simulink model "TRUAV_Dynamics_from_GTRS_trim"  (R2022b)
settings: Solver=ode4  StartTime=0.0  StopTime=3  FixedStep=0.004  RelTol=1e-3
values from neighbouring files (symbols this model uses):
  a_sound = 1116.45    [init_0_GTRS_data_Run_this_file.m]
  alpha_F_rad = alpha_F_deg * (pi/180)    [init_Vetical_2_Table.m]
  alpha_F_rad_table = alpha_F_table * (pi/180)    [init_Fuselage_Aero_Table.m]
  alpha_H_rad = alpha_H_deg * (pi/180)    [init_Horizontal_Table.m]
  alpha_HD_rad = alpha_HD_deg * (pi/180)    [init_Horizontal_C_D_Table.m]
  alpha_r0 = 0    [init_0_GTRS_data_Run_this_file.m]
  alpha_WF_epsilon_M_rad = alpha_WF_deg * pi/180    [init_WingWake_Deflection_Table.m]
  alpha_WS_CL_rad = alpha_WS_CL_deg * (pi/180)    [init_Wing_Slide_Table.m]
  b_w = 32.17    [init_0_GTRS_data_Run_this_file.m]
  beta_F_rad = beta_F_deg * (pi/180)    [init_Vetical_2_Table.m]
  beta_LD_rad_table = beta_LD_table * (pi/180)    [init_Fuselage_Aero_Table.m]
  beta_m_epsilon_M_rad = beta_m_deg * pi/180    [init_WingWake_Deflection_Table.m]
  beta_m_rad_cn = beta_m_deg_cn * pi/180    [init_Wing_Free_Table.m]
  beta_M_rad_table = beta_M_table  * (pi/180)    [init_Fuselage_Aero_Table.m]
  beta_m_S_rad = beta_m_S_deg * (pi/180)    [init_Vetical_2_Table.m]
  beta_m_WS_CL_rad = beta_m_WS_CL_deg * (pi/180)    [init_Wing_Slide_Table.m]
  beta_rad_brk = beta_KBR_rad    [init_Vetical_2_Table.m]
  beta_v_rad = beta_v_deg * (pi/180)    [init_Vetical_1_Table.m]
  beta_vD_rad = beta_vD_deg * (pi/180)    [init_Vetical_1_Table.m]
  beta_WF_Cl_rad = beta_W_deg * (pi/180)    [init_Wing_Free_Table.m]
  beta_WF_CL_rad = beta_CL_deg * (pi/180)    [init_Wing_Free_Table.m]
  beta_YlN_rad_table = beta_YlN_table * (pi/180)    [init_Fuselage_Aero_Table.m]
  c_HW = 3.92    [init_0_GTRS_data_Run_this_file.m]
  C_l_beta_CLwp_table = [ ... (first row only)    [init_Wing_Free_Table.m]
  C_l_beta_pro_CLwp_table = [ ... (first row only)    [init_Wing_Free_Table.m]
  C_L_delta_a_table = [0.00316, 0.00396, 0.00476, 0]    [init_Wing_Free_Table.m]
  C_LHB = -0.00422    [init_0_GTRS_data_Run_this_file.m]
  C_lp_C_LWP = -0.774    [init_0_GTRS_data_Run_this_file.m]
  C_m_wp_table = [ ... (first row only)    [init_Wing_Free_Table.m]
  C_MHA = 0    [init_0_GTRS_data_Run_this_file.m]
  C_MHO = 0    [init_0_GTRS_data_Run_this_file.m]
  c_R = 14/12    (= 1.16666666667)    [init_0_GTRS_data_Run_this_file.m]
  c_w = 5.225    [init_0_GTRS_data_Run_this_file.m]
  C_Y_beta = 0    [init_0_GTRS_data_Run_this_file.m]
  CD0_high_Mach_data = [0.0177, 0.0178, 0.0179, 0.0405]    [init_Wing_Free_Table.m]
  CD_4D_table = zeros(49, 4, 2, 4)    [init_Wing_Slide_Table.m]
  CDH_2D_table = zeros(length(alpha_HD_deg), length(mach_vec))    [init_Horizontal_C_D_Table.m]
  CDV_2D_table = zeros(length(beta_vD_deg), length(mach_vec))    [init_Vetical_1_Table.m]
  CL_4D_table = zeros(49, 4, 2, 4)    [init_Wing_Slide_Table.m]
  CLH_3D_table = zeros(length(alpha_H_deg), length(delta_e_deg), length(mach_vec))    [init_Horizontal_Table.m]
  CYV_3D_table = zeros(length(beta_v_deg), length(delta_r_deg), length(mach_vec))    [init_Vetical_1_Table.m]
  D_alpha_table = [D_part1, D_part2, D_part3, D_part4]    [init_Fuselage_Aero_Table.m]
  D_beta_table = [ fliplr(D_beta_half(2:end)),  D_beta_half]    [init_Fuselage_Aero_Table.m]
  D_ke = 0.24    [init_0_GTRS_data_Run_this_file.m]
  D_Kr = 0.24    [init_0_GTRS_data_Run_this_file.m]    (also in init_Vetical_1_Table.m)
  DBFO = -1.56    [init_0_GTRS_data_Run_this_file.m]
  delta_e_rad = delta_e_deg * (pi/180)    [init_Horizontal_Table.m]
  delta_r_deg = [-20, -15, 0, 15, 20]    [init_Vetical_1_Table.m]
  DLANG = -0.5    [init_0_GTRS_data_Run_this_file.m]
  epsilon_W_table = permute(epsilon_W_3D, [3, 1, 2])    [init_WingWake_Deflection_Table.m]
  flap_rad = flap_deg * (pi/180)    [init_Wing_Free_Table.m]    (also in init_Wing_Slide_Table.m)
  ft2m = 0.3048    [init_0_GTRS_data_Run_this_file.m]
  h_HW = [-0.5838, 0.01158, 0.5967, 0.002547,-2.2519]    [init_0_GTRS_data_Run_this_file.m]
  I_b = 102.5    [init_0_GTRS_data_Run_this_file.m]
  i_H = 0    [init_0_GTRS_data_Run_this_file.m]
  i_v = 0    [init_0_GTRS_data_Run_this_file.m]
  i_w = 0    [init_0_GTRS_data_Run_this_file.m]
  in2ft = 1/12    (= 0.0833333333333)    [init_0_GTRS_data_Run_this_file.m]
  Ixx = 52795    [init_0_GTRS_data_Run_this_file.m]
  Ixz = 1234    [init_0_GTRS_data_Run_this_file.m]
  Iyy = 21360    [init_0_GTRS_data_Run_this_file.m]
  Izz = 66335    [init_0_GTRS_data_Run_this_file.m]
  K1delta_data = [ ... (first row only)    [init_Wing_Free_Table.m]
  K_coeffs = [1.6 0]    [init_0_GTRS_data_Run_this_file.m]
  K_FWDF = -0.0035    [init_0_GTRS_data_Run_this_file.m]
  K_FWO = 1.4    [init_0_GTRS_data_Run_this_file.m]
  K_HNU = 0.8    [init_0_GTRS_data_Run_this_file.m]
  K_vNU = 1    [init_Vetical_1_Table.m]
  KBR_table = KBR_table_full    [init_Vetical_2_Table.m]
  Kn_delta_data = [ ... (first row only)    [init_Wing_Free_Table.m]
  Kno_delta_data = [ ... (first row only)    [init_Wing_Free_Table.m]
  L_alpha_table = [L_part1, L_part2, L_part3, L_part4]    [init_Fuselage_Aero_Table.m]
  L_beta_table = [ fliplr(L_beta_half(2:end)),  L_beta_half]    [init_Fuselage_Aero_Table.m]
  l_beta_table = [l_beta_neg, l_beta_pos]    [init_Fuselage_Aero_Table.m]
  L_n = 4.667    [init_0_GTRS_data_Run_this_file.m]
  lambda_w = -6.5*deg2rad    (= -0.11344640138)    [init_0_GTRS_data_Run_this_file.m]
  LBFO = -7.23    [init_0_GTRS_data_Run_this_file.m]
  LLANG = 0    [init_0_GTRS_data_Run_this_file.m]
  m2ft = 1/ft2m    (= 3.28083989501)    [init_0_GTRS_data_Run_this_file.m]
  M_alpha_table = [M_part1, M_part2, M_part3, M_part4]    [init_Fuselage_Aero_Table.m]
  M_beta_table = [ fliplr(M_beta_half(2:end)), M_beta_half]    [init_Fuselage_Aero_Table.m]
  Mach_brk = [0.2, 0.4, 0.5, 0.6]    [init_Wing_Free_Table.m]
  mach_vec = [0.2, 0.4, 0.5, 0.6]    [init_Horizontal_C_D_Table.m]    (also in init_Horizontal_Table.m; init_Vetical_1_Table.m)
  mass = 403.7    [init_0_GTRS_data_Run_this_file.m]
  mast_rad = mast_deg * pi/180    [init_Wing_Free_Table.m]
  MBFO = 66.5    [init_0_GTRS_data_Run_this_file.m]
  Mn_X_ke = [0 0.2 0.4 0.5 0.6 0.7]    [init_Horizontal_Table.m]
  N_beta_table = [N_beta_neg, N_beta_pos]    [init_Fuselage_Aero_Table.m]
  pos_x_CG = 300    [init_0_GTRS_data_Run_this_file.m]
  pos_x_H = 300    [init_0_GTRS_data_Run_this_file.m]
  pos_x_HW = 560    [init_0_GTRS_data_Run_this_file.m]
  pos_x_Nac = 291.7    [init_0_GTRS_data_Run_this_file.m]
  pos_x_V = 570    [init_0_GTRS_data_Run_this_file.m]
  pos_x_W = 291.7    [init_0_GTRS_data_Run_this_file.m]
  pos_y_CG = 0    [init_0_GTRS_data_Run_this_file.m]
  pos_y_H = 193    [init_0_GTRS_data_Run_this_file.m]
  pos_y_HW = 0    [init_0_GTRS_data_Run_this_file.m]
  pos_y_Nac = 193    [init_0_GTRS_data_Run_this_file.m]
  pos_y_V = 115.69    [init_0_GTRS_data_Run_this_file.m]
  pos_y_W = 96.6    [init_0_GTRS_data_Run_this_file.m]
  pos_z_CG = 81.65    [init_0_GTRS_data_Run_this_file.m]
  pos_z_H = 100    [init_0_GTRS_data_Run_this_file.m]
  pos_z_HW = 103    [init_0_GTRS_data_Run_this_file.m]
  pos_z_Nac = 118    [init_0_GTRS_data_Run_this_file.m]
  pos_z_V = 77    [init_0_GTRS_data_Run_this_file.m]
  pos_z_W = 96    [init_0_GTRS_data_Run_this_file.m]
  R = 12.5    [init_0_GTRS_data_Run_this_file.m]
  rho = 0.002376    [init_0_GTRS_data_Run_this_file.m]
  s_HW = 50.25    [init_0_GTRS_data_Run_this_file.m]
  S_max = 56    [init_0_GTRS_data_Run_this_file.m]
  S_v = 20.25    [init_0_GTRS_data_Run_this_file.m]
  S_w = 181    [init_0_GTRS_data_Run_this_file.m]
  Sidewash_4D = zeros(length(alpha_F_deg), length(beta_F_deg), length(beta_m_S_deg), length(delta_F_S_deg))    [init_Vetical_2_Table.m]
  slugft2kgm = 1.35582    [init_0_GTRS_data_Run_this_file.m]
  tau_e = 0.518    [init_0_GTRS_data_Run_this_file.m]
  tau_r = 0.27    [init_0_GTRS_data_Run_this_file.m]    (also in init_Vetical_1_Table.m)
  theta_0_R = 0.750    (= 0.75)    [init_0_GTRS_data_Run_this_file.m]
  theta_0_W = 1.187    [init_0_GTRS_data_Run_this_file.m]
  theta_twist = -41*deg2rad    (= -0.715584993318)    [init_0_GTRS_data_Run_this_file.m]
  u_max = 1181/12    (= 98.4166666667)    [init_0_GTRS_data_Run_this_file.m]
  ... (+3 more)
undefined symbols (not defined in the file or in its folder): beta_m_rad, F, Light, MIL, sigbuilder_block, tilt_cmd
libraries: simulink x2, sharedtransform x2, aerolibasang x2, aerolibwind2 x1
(part 1 of 4)
settings Model: PacingRate=10  Creator=57178  LastModifiedBy=57178

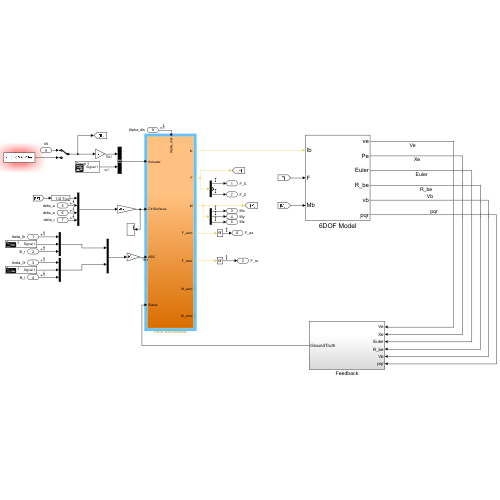
[thumbnail: Simulink's stored preview of the top-level diagram]
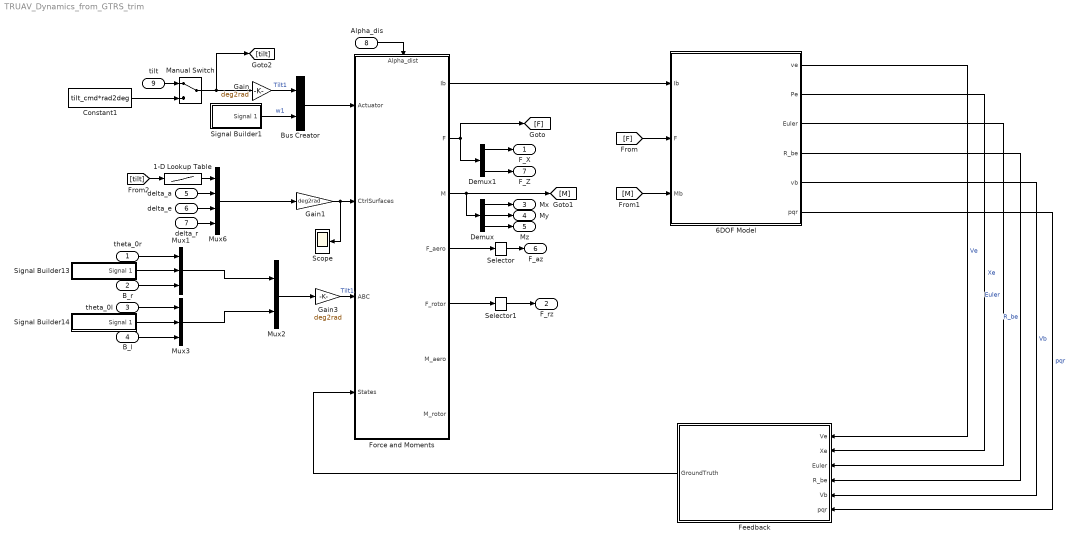
== system TRUAV_Dynamics_from_GTRS_trim ==
  theta_0r : Inport
  B_r : Inport  Port=2
  theta_0l : Inport  Port=3
  B_l : Inport  Port=4
  delta_a : Inport  Port=5
  delta_e : Inport  Port=6
  delta_r : Inport  Port=7
  Alpha_dis : Inport  Port=8
  tilt : Inport  Port=9
  1-D Lookup Table : Lookup_n-D  NumberOfTableDimensions=1  BreakpointsForDimension1=[0, 15, 30, 60, 90]  Table=[75, 75, 50, 10, 0]  InternalRulePriority=Speed  RndMeth=Simplest
  6DOF Model : Subsystem
  Bus Creator : BusCreator  Inputs=2
  Constant1 : Constant  Value=tilt_cmd*rad2deg
  Demux : Demux  Outputs=3
  Demux1 : Demux  Outputs=3
  Feedback : Subsystem
  Force and Moments : Subsystem
      settings: PortSchema="{\"entries\":[{\"content\":{\"sides\":[{\"content\":{\"connectorIds\":[\"In1\",\"In2\",\"In3\",\"In4\"]},\"type\":\"ConnectorPlacement.EquallySpacedRectSide\",\"uuid\":\"14175658-dd1e-49e4-b43b-ea4e1e064656\"},{\"content\":{\"connectorIds\":[\"Out1\",\"Out2\",\"Out3\",\"Out4\",\"Out5\",\"Out6\",\"Out7\"],\"side\":\"RIGHT\"},\"type\":\"ConnectorPlacement.EquallySpacedRectSide\",\"uuid\":\"2cac6120-f4ef-4ea4-82cf-37ab6ff67795\"},{\"content\":{\"connectorIds\":[\"In5\"],\"side\":\"TOP\"},\"type\":\"ConnectorPlacement.EquallySpacedRectSide\",\"uuid\":\"384cf1cc-0caa-4cb0-88f0-d3cb4556450a\"}]},\"type\":\"ConnectorPlacement.EquallySpacedConnector\",\"uuid\":\"6851ebde-8421-46a5-9721-7873d89ee264\"}],\"packageUris\":[\"http://schema.mathworks.com/mf0/Connector/R2020b\"],\"version\":\"1.0\"}"
  Gain : Gain  Gain=deg2rad
  Gain1 : Gain  Gain=deg2rad
  Gain3 : Gain  Gain=deg2rad
  Manual Switch : ManualSwitch
  Mux1 : Mux  Inputs=3
  Mux2 : Mux  Inputs=2
  Mux3 : Mux  Inputs=3
  Mux6 : Mux
  Scope : Scope
  Selector : Selector  InputPortWidth=3  IndexOptions=Index vector (dialog)  Indices=[3]  OutputSizes=1
  Selector1 : Selector  InputPortWidth=3  IndexOptions=Index vector (dialog)  Indices=[3]  OutputSizes=1
  Signal Builder1 : Subsystem  Tag=STV Subsys  LoadFcn=sigbuilder_block('load');  StartFcn=sigbuilder_block('start');  StopFcn=sigbuilder_block('stop');  ClipboardFcn=sigbuilder_block('clipboard');  mask(Sigbuilder block){tuvar=[0:10]}
      mask help: Simulink:masks:SigbuilderBlock_MD
      mask init:
      | if ~strcmp(get_param(bdroot(gcbh),'SimulationStatus'),'stopped') tuvar = sigbuilder_block('maskInit'); end
      settings: CopyFcn=sigbuilder_block('copy');  DeleteFcn=sigbuilder_block('delete');  ModelCloseFcn=sigbuilder_block('modelClose');  PreSaveFcn=sigbuilder_block('preSave');  PauseFcn=sigbuilder_block('pause');  ContinueFcn=sigbuilder_block('continue');  NameChangeFcn=sigbuilder_block('namechange');  OpenFcn=sigbuilder_block('open',[437.6 199.2 550.4 400 ]);  CloseFcn=sigbuilder_block('close');
      mask Display: plot(0, 0, 100, 100,[2, 2, 32, 32, 2], [68, 8, 8, 68, 68],[32, 2], [38, 38], [32, 19, 2],[53, 60, 44], [32, 17, 17, 2],[16, 16, 31, 31]);txt = getActiveGroup(gcbh);text(2, 100, txt,'verticalAlignment', 'top');
  Signal Builder13 : Subsystem  Tag=STV Subsys  LoadFcn=sigbuilder_block('load');  StartFcn=sigbuilder_block('start');  StopFcn=sigbuilder_block('stop');  ClipboardFcn=sigbuilder_block('clipboard');  mask(Sigbuilder block){tuvar=[0:10]}
      mask help: Simulink:masks:SigbuilderBlock_MD
      mask init:
      | if ~strcmp(get_param(bdroot(gcbh),'SimulationStatus'),'stopped') tuvar = sigbuilder_block('maskInit'); end
      settings: CopyFcn=sigbuilder_block('copy');  DeleteFcn=sigbuilder_block('delete');  ModelCloseFcn=sigbuilder_block('modelClose');  PreSaveFcn=sigbuilder_block('preSave');  PauseFcn=sigbuilder_block('pause');  ContinueFcn=sigbuilder_block('continue');  NameChangeFcn=sigbuilder_block('namechange');  OpenFcn=sigbuilder_block('open',[-1344 -173.143 550.286 399.857 ]);  CloseFcn=sigbuilder_block('close');
      mask Display: plot(0, 0, 100, 100,[2, 2, 32, 32, 2], [68, 8, 8, 68, 68],[32, 2], [38, 38], [32, 19, 2],[53, 60, 44], [32, 17, 17, 2],[16, 16, 31, 31]);txt = getActiveGroup(gcbh);text(2, 100, txt,'verticalAlignment', 'top');
  Signal Builder14 : Subsystem  Tag=STV Subsys  LoadFcn=sigbuilder_block('load');  StartFcn=sigbuilder_block('start');  StopFcn=sigbuilder_block('stop');  ClipboardFcn=sigbuilder_block('clipboard');  mask(Sigbuilder block){tuvar=[0:10]}
      mask help: Simulink:masks:SigbuilderBlock_MD
      mask init:
      | if ~strcmp(get_param(bdroot(gcbh),'SimulationStatus'),'stopped') tuvar = sigbuilder_block('maskInit'); end
      settings: CopyFcn=sigbuilder_block('copy');  DeleteFcn=sigbuilder_block('delete');  ModelCloseFcn=sigbuilder_block('modelClose');  PreSaveFcn=sigbuilder_block('preSave');  PauseFcn=sigbuilder_block('pause');  ContinueFcn=sigbuilder_block('continue');  NameChangeFcn=sigbuilder_block('namechange');  OpenFcn=sigbuilder_block('open',[-1344 -173.143 550.286 399.857 ]);  CloseFcn=sigbuilder_block('close');
      mask Display: plot(0, 0, 100, 100,[2, 2, 32, 32, 2], [68, 8, 8, 68, 68],[32, 2], [38, 38], [32, 19, 2],[53, 60, 44], [32, 17, 17, 2],[16, 16, 31, 31]);txt = getActiveGroup(gcbh);text(2, 100, txt,'verticalAlignment', 'top');
  F_X : Outport
  F_rz : Outport  Port=2
  Mx : Outport  Port=3
  My : Outport  Port=4
  Mz : Outport  Port=5
  F_az : Outport  Port=6
  F_Z : Outport  Port=7
  wires:
  6DOF Model/5(vb) -> Feedback/5(Vb)  "Vb"
  6DOF Model/4(R_be) -> Feedback/4(R_be)  "R_be"
  6DOF Model/2(Pe) -> Feedback/2(Xe)  "Xe"
  [M] -> 6DOF Model/3(Mb)
  [F] -> 6DOF Model/2(F)
  6DOF Model/3(Euler) -> Feedback/3(Euler)  "Euler"
  6DOF Model/6(pqr) -> Feedback/6(pqr)  "pqr"
  Feedback/1(GroundTruth) -> Force and Moments/4(States)
  6DOF Model/1(ve) -> Feedback/1(Ve)  "Ve"
  Force and Moments/2(F) -> Demux1/1, [F]
  Force and Moments/3(M) -> Demux/1, [M]
  Gain/1 -> Bus Creator/1  "Tilt1"
  Signal Builder1/1(Signal 1) -> Bus Creator/2  "w1"
  Bus Creator/1 -> Force and Moments/1(Actuator)
  Mux6/1 -> Gain1/1
  Mux2/1 -> Gain3/1
  Manual Switch/1 -> [tilt], Gain/1
  Gain3/1 -> Force and Moments/3(ABC)  "Tilt1"
  Gain1/1 -> Scope/1, Force and Moments/2(CtrlSurfaces)
  Force and Moments/1(Ib) -> 6DOF Model/1(Ib)
  theta_0r/1 -> Mux1/1
  Signal Builder13/1(Signal 1) -> Mux1/2
  B_r/1 -> Mux1/3
  theta_0l/1 -> Mux3/1
  Signal Builder14/1(Signal 1) -> Mux3/2
  B_l/1 -> Mux3/3
  Mux1/1 -> Mux2/1
  Mux3/1 -> Mux2/2
  1-D Lookup Table/1 -> Mux6/1
  delta_r/1 -> Mux6/4
  delta_e/1 -> Mux6/3
  delta_a/1 -> Mux6/2
  Demux/1 -> Mx/1
  Demux/3 -> Mz/1
  Demux/2 -> My/1
  Demux1/1 -> F_X/1
  Demux1/3 -> F_Z/1
  Alpha_dis/1 -> Force and Moments/5(Alpha_dist)
  Force and Moments/4(F_aero) -> Selector/1
  Selector/1 -> F_az/1
  Selector1/1 -> F_rz/1
  [tilt] -> 1-D Lookup Table/1
  Force and Moments/5(F_rotor) -> Selector1/1
  Constant1/1 -> Manual Switch/2
  tilt/1 -> Manual Switch/1

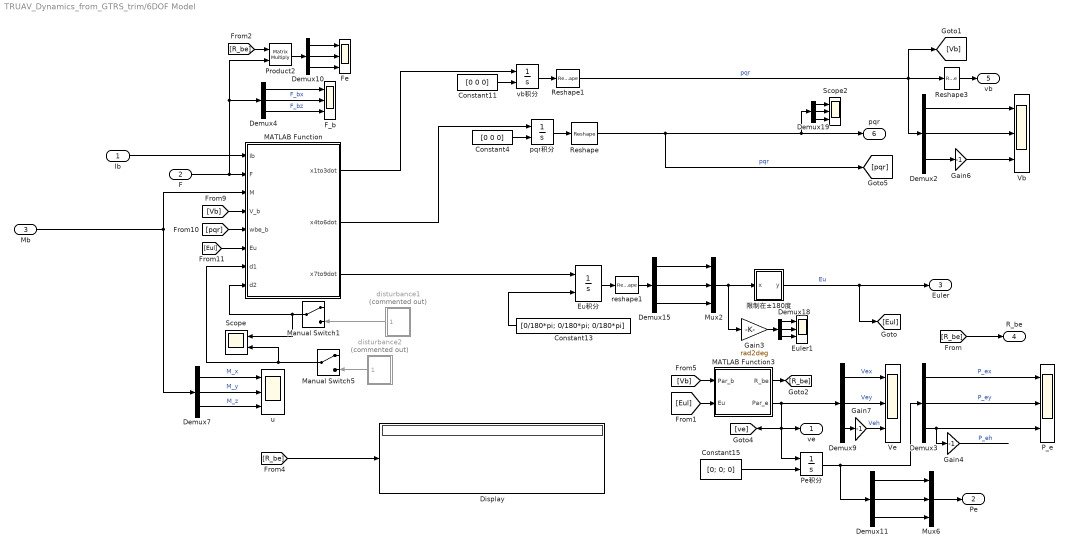
== system TRUAV_Dynamics_from_GTRS_trim/6DOF Model ==
  Ib : Inport
  F : Inport  Port=2
  Mb : Inport  Port=3
  Constant11 : Constant  Value=[0 0 0]
  Constant13 : Constant  Value=[0/180*pi; 0/180*pi; 0/180*pi]
  Constant15 : Constant  Value=[0; 0; 0]
  Constant4 : Constant  Value=[0 0 0]
  Demux{2..4,7,9..11,15,18..19} (10 alike) : Demux  Outputs=3
  Display : Display
  Euler1 : Scope  NumInputPorts=3
  Eu积分 : Integrator  InitialConditionSource=external
  F_b : Scope  NumInputPorts=3
  Fe : Scope  NumInputPorts=3
  Gain3 : Gain  Gain=rad2deg
  Gain4 : Gain  Gain=-1
  Gain6 : Gain  Gain=-1
  Gain7 : Gain  Gain=-1
  MATLAB Function : MATLAB Function  TreatAsAtomicUnit=on
  MATLAB Function3 : MATLAB Function  TreatAsAtomicUnit=on
  Manual Switch1 : ManualSwitch
  Manual Switch5 : ManualSwitch
  Mux2 : Mux  Inputs=3
  Mux6 : Mux  Inputs=3
  P_e : Scope  NumInputPorts=3
  Pe积分 : Integrator  InitialConditionSource=external
  Product2 : Product  Multiplication=Matrix(*)
  Reshape : Reshape  OutputDimensionality=Customize  OutputDimensions=[3,1]
  Reshape1 : Reshape  OutputDimensionality=Customize  OutputDimensions=[3,1]
  Reshape3 : Reshape  OutputDimensionality=Column vector (2-D)
  Scope : Scope  NumInputPorts=2
  Scope2 : Scope  NumInputPorts=3
  Vb : Scope  NumInputPorts=3
  Ve : Scope  NumInputPorts=3
  disturbance1 : Subsystem  Commented=on
  disturbance2 : Subsystem  Commented=on
  pqr积分 : Integrator  InitialConditionSource=external
  reshape1 : Reshape  OutputDimensionality=Customize  OutputDimensions=[3,1]
  u : Scope  NumInputPorts=3
  vb积分 : Integrator  InitialConditionSource=external
  限制在±180度 : MATLAB Function  TreatAsAtomicUnit=on
  ve : Outport
  Pe : Outport  Port=2
  Euler : Outport  Port=3  VectorParamsAs1DForOutWhenUnconnected=off
  R_be : Outport  Port=4  VectorParamsAs1DForOutWhenUnconnected=off
  vb : Outport  Port=5  VectorParamsAs1DForOutWhenUnconnected=off
  pqr : Outport  Port=6  VectorParamsAs1DForOutWhenUnconnected=off
  wires:
  Demux3/3 -> P_e/3, Gain4/1
  Demux3/1 -> P_e/1  "P_ex"
  [Eul] -> MATLAB Function3/2(Eu)
  MATLAB Function3/2(Par_e) -> Pe积分/1, [ve], ve/1, Demux9/1
  Demux9/3 -> Gain7/1
  Demux9/1 -> Ve/1  "Vex"
  Demux9/2 -> Ve/2  "Vey"
  Mb/1 -> MATLAB Function/3(M), Demux7/1
  Demux7/3 -> u/3  "M_z"
  Demux7/1 -> u/1  "M_x"
  Demux7/2 -> u/2  "M_y"
  限制在±180度/1(y) -> [Eul], Euler/1  "Eu"
  Manual Switch1/1 -> MATLAB Function/8(d2), Scope/1
  Demux4/1 -> F_b/1  "F_bx"
  Demux4/2 -> F_b/2
  Demux4/3 -> F_b/3  "F_bz"
  Demux2/3 -> Gain6/1
  Demux2/2 -> Vb/2
  Demux2/1 -> Vb/1
  Demux15/3 -> Mux2/3
  Demux15/1 -> Mux2/1
  Mux2/1 -> Gain3/1, 限制在±180度/1(x)
  pqr积分/1 -> Reshape/1
  MATLAB Function/1(x1to3dot) -> vb积分/1
  reshape1/1 -> Demux15/1
  Eu积分/1 -> reshape1/1
  MATLAB Function/3(x7to9dot) -> Eu积分/1
  Constant4/1 -> pqr积分/2
  Constant11/1 -> vb积分/2
  vb积分/1 -> Reshape1/1
  disturbance1/1(Out1) -> Manual Switch1/2
  Demux18/2 -> Euler1/2
  Demux18/3 -> Euler1/3
  Demux18/1 -> Euler1/1
  Gain3/1 -> Demux18/1
  Demux19/3 -> Scope2/3
  Demux19/1 -> Scope2/1
  Demux19/2 -> Scope2/2
  Constant15/1 -> Pe积分/2
  MATLAB Function3/1(R_be) -> [R_be]
  [R_be] -> R_be/1
  Demux3/2 -> P_e/2  "P_ey"
  Gain4/1 -> ?  "P_eh"
  [R_be] -> Display/1
  MATLAB Function/2(x4to6dot) -> pqr积分/1
  Constant13/1 -> Eu积分/2
  [Vb] -> MATLAB Function3/1(Par_b)
  Mux6/1 -> Pe/1
  Demux11/2 -> Mux6/2
  Pe积分/1 -> Demux11/1, Demux3/1
  Demux11/3 -> Mux6/3
  Demux11/1 -> Mux6/1
  Demux15/2 -> Mux2/2
  Demux10/3 -> Fe/3
  Product2/1 -> Demux10/1
  Demux10/2 -> Fe/2
  Demux10/1 -> Fe/1
  [R_be] -> Product2/1
  F/1 -> MATLAB Function/2(F), Product2/2, Demux4/1
  [Vb] -> MATLAB Function/4(V_b)
  [pqr] -> MATLAB Function/5(wbe_b)
  [Eul] -> MATLAB Function/6(Eu)
  Manual Switch5/1 -> MATLAB Function/7(d1), Scope/2
  Gain6/1 -> Vb/3
  Gain7/1 -> Ve/3  "Veh"
  Ib/1 -> MATLAB Function/1(Ib)
  disturbance2/1(Out1) -> Manual Switch5/2
  Reshape1/1 -> Demux2/1, Reshape3/1, [Vb]  "pqr"
  Reshape3/1 -> vb/1
  Reshape/1 -> Demux19/1, pqr/1, [pqr]  "pqr"

== system TRUAV_Dynamics_from_GTRS_trim/Feedback ==
  Ve : Inport
  Xe : Inport  Port=2
  Euler : Inport  Port=3
  R_be : Inport  Port=4
  Vb : Inport  Port=5
  pqr : Inport  Port=6
  Direction Cosine Matrix to Quaternions : sharedtransform/Direction Cosine Matrix  to Quaternions  aMode=0  action=None  tolerance=eps(2)
      settings: LibrarySourceBlock=|
      | aerolibtransform2/Direction Cosine Matrix
      | to Quaternions
  MATLAB Function1 : MATLAB Function  TreatAsAtomicUnit=on
  Reshape : Reshape  OutputDimensionality=Column vector (2-D)
  Reshape1 : Reshape  OutputDimensionality=Column vector (2-D)
  Selector : Selector  InputPortWidth=3  IndexOptions=Index vector (dialog)  Indices=[3 2 1]  OutputSizes=1
  Transpose : Math  Operator=transpose
  Bus Element Out : Outport  PortName=GroundTruth  Element=course
  Bus Element Out1 : Outport  PortName=GroundTruth  Element=gndspeed
  Bus Element Out3 : Outport  PortName=GroundTruth  Element=Xe
  Bus Element Out4 : Outport  PortName=GroundTruth  Element=Ve
  Bus Element Out7 : Outport  PortName=GroundTruth  Element=R_be
  Bus Element Out8 : Outport  PortName=GroundTruth  Element=q
  Bus Element Out9 : Outport  PortName=GroundTruth  Element=pqr
  Bus Element Out6 : Outport  PortName=GroundTruth  Element=Vb
  Bus Element Out5 : Outport  PortName=GroundTruth  Element=Euler
  Bus Element Out13 : Outport  PortName=GroundTruth  Element=ypr
  Bus Element Out14 : Outport  PortName=GroundTruth  Element=Ve_ground
  wires:
  Reshape1/1 -> Bus Element Out6/1
  Reshape/1 -> Bus Element Out5/1, Selector/1
  Selector/1 -> Bus Element Out13/1
  pqr/1 -> Bus Element Out9/1
  Direction Cosine Matrix to Quaternions/1 -> Bus Element Out8/1  "q"
  Vb/1 -> Reshape1/1
  Euler/1 -> Reshape/1
  Xe/1 -> Bus Element Out3/1
  MATLAB Function1/2(gndSpeed) -> Bus Element Out1/1  "gndspeed"
  MATLAB Function1/1(course) -> Bus Element Out/1  "course"
  Ve/1 -> MATLAB Function1/1(vxyz), Bus Element Out4/1, Bus Element Out14/1
  R_be/1 -> Transpose/1, Bus Element Out7/1
  Transpose/1 -> Direction Cosine Matrix to Quaternions/1

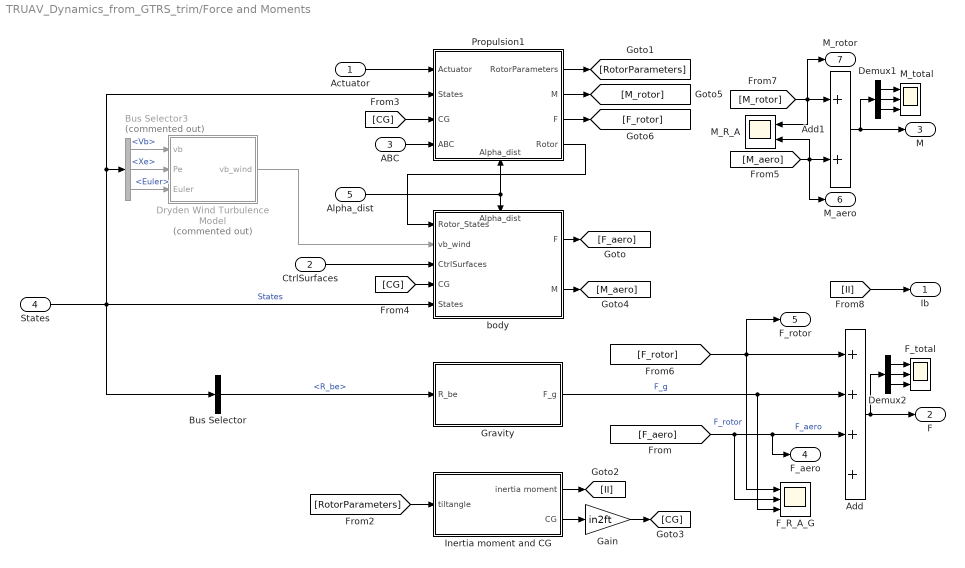
== system TRUAV_Dynamics_from_GTRS_trim/Force and Moments ==
  Actuator : Inport
  CtrlSurfaces : Inport  Port=2
  ABC : Inport  Port=3
  States : Inport  Port=4
  Alpha_dist : Inport  Port=5
  Add : Sum  Inputs=++++
  Add1 : Sum
  Bus Selector : BusSelector  OutputSignals=R_be
  Bus Selector3 : BusSelector  Commented=on  OutputSignals=Vb,Xe,Euler
  Demux1 : Demux  Outputs=3
  Demux2 : Demux  Outputs=3
  "Dryden Wind Turbulence Model " : Subsystem  Commented=on
  F_R_A_G : Scope  NumInputPorts=3
  F_total : Scope  NumInputPorts=3
  Gain : Gain  Gain=in2ft
  Gravity : Subsystem
  Inertia moment and CG : Subsystem
  M_R_A : Scope  NumInputPorts=2
  M_total : Scope  NumInputPorts=3
  Propulsion1 : Subsystem
      settings: PortSchema="{\"entries\":[{\"content\":{\"sides\":[{\"content\":{\"connectorIds\":[\"In1\",\"In2\",\"In3\",\"In4\"]},\"type\":\"ConnectorPlacement.EquallySpacedRectSide\",\"uuid\":\"6f2dbf48-690a-489c-8000-4c6cd685a3c0\"},{\"content\":{\"connectorIds\":[\"Out1\",\"Out2\",\"Out3\",\"Out4\"],\"side\":\"RIGHT\"},\"type\":\"ConnectorPlacement.EquallySpacedRectSide\",\"uuid\":\"c26906ca-dfe8-4bd8-a446-638a7a033ba1\"},{\"content\":{\"connectorIds\":[],\"side\":\"TOP\"},\"type\":\"ConnectorPlacement.EquallySpacedRectSide\",\"uuid\":\"7c8468f6-8fb2-4195-8877-8a49a6dfa1f5\"},{\"content\":{\"connectorIds\":[\"In5\"],\"side\":\"BOTTOM\"},\"type\":\"ConnectorPlacement.EquallySpacedRectSide\",\"uuid\":\"9f190dd0-766f-495f-83f9-cb048c56ad4a\"}]},\"type\":\"ConnectorPlacement.EquallySpacedConnector\",\"uuid\":\"be6e6569-2cab-4e42-86d9-8b4e7133f4ae\"}],\"packageUris\":[\"http://schema.mathworks.com/mf0/Connector/R2020b\"],\"version\":\"1.0\"}"
  body : Subsystem
      settings: PortSchema="{\"entries\":[{\"content\":{\"sides\":[{\"content\":{\"connectorIds\":[\"In1\",\"In2\",\"In3\",\"In4\",\"In5\"]},\"type\":\"ConnectorPlacement.EquallySpacedRectSide\",\"uuid\":\"57bbf977-6343-4159-b754-e5d2e9fd81d9\"},{\"content\":{\"connectorIds\":[\"Out1\",\"Out2\"],\"side\":\"RIGHT\"},\"type\":\"ConnectorPlacement.EquallySpacedRectSide\",\"uuid\":\"304a29c9-3542-4502-b32f-72f6699ccbb9\"},{\"content\":{\"connectorIds\":[\"In6\"],\"side\":\"TOP\"},\"type\":\"ConnectorPlacement.EquallySpacedRectSide\",\"uuid\":\"a47e5583-e12a-44fe-beb4-06c0064b8ef5\"},{\"content\":{\"connectorIds\":[],\"side\":\"BOTTOM\"},\"type\":\"ConnectorPlacement.EquallySpacedRectSide\",\"uuid\":\"46911a4c-96f8-437e-85a1-c5a709ead67b\"}]},\"type\":\"ConnectorPlacement.EquallySpacedConnector\",\"uuid\":\"5ab3fb2f-b501-478f-a319-bc831e44ee3d\"}],\"packageUris\":[\"http://schema.mathworks.com/mf0/Connector/R2020b\"],\"version\":\"1.0\"}"
  Ib : Outport
  F : Outport  Port=2
  M : Outport  Port=3
  F_aero : Outport  Port=4
  F_rotor : Outport  Port=5
  M_aero : Outport  Port=6
  M_rotor : Outport  Port=7
  wires:
  Gravity/1(F_g) -> F_R_A_G/3, Add/2  "F_g"
  States/1 -> Bus Selector/1, body/5(States), Propulsion1/2(States), Bus Selector3/1  "States"
  [F_aero] -> F_R_A_G/2, F_aero/1, Add/3  "F_aero"
  Bus Selector3/2 -> "Dryden Wind Turbulence Model "/2(Pe)  "<Xe>"
  Bus Selector3/3 -> "Dryden Wind Turbulence Model "/3(Euler)  "<Euler>"
  Bus Selector/1 -> Gravity/1(R_be)  "<R_be>"
  [RotorParameters] -> Inertia moment and CG/1(tiltangle)
  Inertia moment and CG/1(inertia moment) -> [II]
  Inertia moment and CG/2(CG) -> Gain/1
  [CG] -> Propulsion1/3(CG)
  Propulsion1/1(RotorParameters) -> [RotorParameters]
  Actuator/1 -> Propulsion1/1(Actuator)
  [CG] -> body/4(CG)
  Gain/1 -> [CG]
  CtrlSurfaces/1 -> body/3(CtrlSurfaces)
  Propulsion1/4(Rotor) -> body/1(Rotor_States)
  body/1(F) -> [F_aero]
  body/2(M) -> [M_aero]
  Propulsion1/2(M) -> [M_rotor]
  Propulsion1/3(F) -> [F_rotor]
  [F_rotor] -> Add/1, F_rotor/1, F_R_A_G/1  "F_rotor"
  [M_rotor] -> Add1/1, M_rotor/1, M_R_A/1
  [II] -> Ib/1
  ABC/1 -> Propulsion1/4(ABC)
  Demux1/2 -> M_total/2
  Demux1/3 -> M_total/3
  Demux1/1 -> M_total/1
  Add1/1 -> M/1, Demux1/1
  Demux2/1 -> F_total/1
  Demux2/3 -> F_total/3
  Demux2/2 -> F_total/2
  Add/1 -> F/1, Demux2/1
  Alpha_dist/1 -> Propulsion1/5(Alpha_dist), body/6(Alpha_dist)
  [M_aero] -> Add1/2, M_aero/1, M_R_A/2
  Bus Selector3/1 -> "Dryden Wind Turbulence Model "/1(vb)  "<Vb>"
  "Dryden Wind Turbulence Model "/1(vb_wind) -> body/2(vb_wind)

== system TRUAV_Dynamics_from_GTRS_trim/Signal Builder1 ==
  Demux : Demux  Tag=STV Demux  Outputs=1
      settings: DisplayOption=none
  FromWs : FromWorkspace  Tag=STV FromWs  VariableName=tuvar
      SigBuilderData=|
      | common.afterFinalStr = 'Extrapolate'
      | common.sampleTime = 0
      | dataSet.timeRange = [0 10]
      | dataSet.name = 'Group 1'
      | sbobj.Groups.Name = 'Group 1'
      | sbobj.Groups.Signals.Name = 'Signal 1'
      | sbobj.Groups.Signals.XData = [0 10]
      | sbobj.Groups.Signals.YData = [589 589]
  Signal 1 : Outport  Tag=STV Outport
  wires:
  FromWs/1 -> Demux/1
  Demux/1 -> Signal 1/1

== system TRUAV_Dynamics_from_GTRS_trim/Signal Builder13 ==
  Demux : Demux  Tag=STV Demux  Outputs=1
      settings: DisplayOption=none
  FromWs : FromWorkspace  Tag=STV FromWs  VariableName=tuvar
      SigBuilderData=|
      | common.afterFinalStr = 'Extrapolate'
      | common.sampleTime = 0
      | dataSet.timeRange = [0 10]
      | dataSet.name = 'Group 1'
      | sbobj.Groups.Name = 'Group 1'
      | sbobj.Groups.Signals.Name = 'Signal 1'
      | sbobj.Groups.Signals.XData = [0 10]
      | sbobj.Groups.Signals.YData = [0 0]
  Signal 1 : Outport  Tag=STV Outport
  wires:
  Demux/1 -> Signal 1/1
  FromWs/1 -> Demux/1

== system TRUAV_Dynamics_from_GTRS_trim/Signal Builder14 ==
  Demux : Demux  Tag=STV Demux  Outputs=1
      settings: DisplayOption=none
  FromWs : FromWorkspace  Tag=STV FromWs  VariableName=tuvar
      SigBuilderData=|
      | common.afterFinalStr = 'Extrapolate'
      | common.sampleTime = 0
      | dataSet.timeRange = [0 10]
      | dataSet.name = 'Group 1'
      | sbobj.Groups.Name = 'Group 1'
      | sbobj.Groups.Signals.Name = 'Signal 1'
      | sbobj.Groups.Signals.XData = [0 10]
      | sbobj.Groups.Signals.YData = [0 0]
  Signal 1 : Outport  Tag=STV Outport
  wires:
  FromWs/1 -> Demux/1
  Demux/1 -> Signal 1/1

== system TRUAV_Dynamics_from_GTRS_trim/6DOF Model/disturbance1 ==
  Add1 : Sum  Commented=on
  Band-Limited White Noise1 : simulink/Sources/Band-Limited White Noise  Commented=on  Cov=[0.1]  Ts=0.1  seed=[23341]
  Clock1 : Clock
  Clock2 : Clock  Commented=on
  Disturb1 : MATLAB Function  TreatAsAtomicUnit=on
  Disturb2 : MATLAB Function  TreatAsAtomicUnit=on
  Disturb4 : MATLAB Function  TreatAsAtomicUnit=on
  Mux8 : Mux  Inputs=3
  Switch : Switch  Commented=on  Criteria=u2 > Threshold  Threshold=12  SaturateOnIntegerOverflow=off  InputSameDT=off
  noise Disturb1 : MATLAB Function  Commented=on  TreatAsAtomicUnit=on
  noise Disturb2 : MATLAB Function  Commented=on  TreatAsAtomicUnit=on
  扰动1 : Scope  NumInputPorts=3
  Out1 : Outport
  wires:
  Disturb2/1(y) -> 扰动1/1, Mux8/1  "d1"
  Clock1/1 -> noise Disturb1/2(t), Disturb4/1(t), noise Disturb2/2(t), Disturb2/1(t), Disturb1/1(t)
  Disturb1/1(y) -> Mux8/2, 扰动1/2  "d2"
  noise Disturb2/1(y) -> Add1/2
  noise Disturb1/1(y) -> Add1/1
  Band-Limited White Noise1/1 -> noise Disturb2/1(n), noise Disturb1/1(n)
  Disturb4/1(y) -> Mux8/3, 扰动1/3  "d3"
  Clock2/1 -> Switch/2
  Mux8/1 -> Out1/1, Switch/3

== system TRUAV_Dynamics_from_GTRS_trim/6DOF Model/disturbance2 ==
  Add1 : Sum  Commented=on
  Band-Limited White Noise1 : simulink/Sources/Band-Limited White Noise  Commented=on  Cov=[0.1]  Ts=0.1  seed=[23341]
  Clock1 : Clock
  Clock2 : Clock  Commented=on
  Disturb1 : MATLAB Function  TreatAsAtomicUnit=on
  Disturb2 : MATLAB Function  TreatAsAtomicUnit=on
  Disturb4 : MATLAB Function  TreatAsAtomicUnit=on
  Mux8 : Mux  Inputs=3
  Switch : Switch  Commented=on  Criteria=u2 > Threshold  Threshold=12  SaturateOnIntegerOverflow=off  InputSameDT=off
  noise Disturb1 : MATLAB Function  Commented=on  TreatAsAtomicUnit=on
  noise Disturb2 : MATLAB Function  Commented=on  TreatAsAtomicUnit=on
  扰动1 : Scope  NumInputPorts=3
  Out1 : Outport
  wires:
  Mux8/1 -> Switch/3, Out1/1
  Clock2/1 -> Switch/2
  Disturb4/1(y) -> Mux8/2, 扰动1/2  "d2"
  Band-Limited White Noise1/1 -> noise Disturb1/1(n), noise Disturb2/1(n)
  noise Disturb1/1(y) -> Add1/1
  noise Disturb2/1(y) -> Add1/2
  Clock1/1 -> Disturb4/1(t), Disturb2/1(t), Disturb1/1(t), noise Disturb2/2(t), noise Disturb1/2(t)
  Disturb2/1(y) -> Mux8/1, 扰动1/1  "d1"
  Disturb1/1(y) -> 扰动1/3, Mux8/3  "d2"

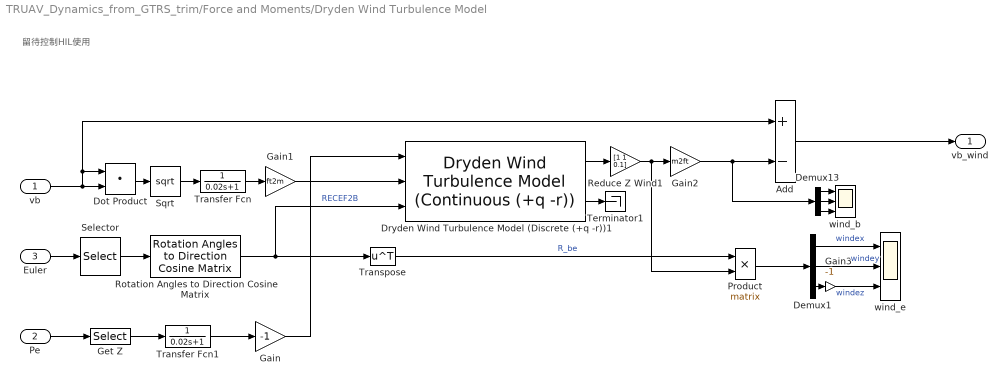
== system TRUAV_Dynamics_from_GTRS_trim/Force and Moments/Dryden Wind Turbulence Model  ==
  note: 留待控制HIL使用
  vb : Inport
  Pe : Inport  Port=2
  Euler : Inport  Port=3
  Add : Sum  Inputs=+-
  Demux1 : Demux  Outputs=3
  Demux13 : Demux  Outputs=3
  Dot Product : DotProduct  OutDataTypeStr=Inherit: Inherit via internal rule
  Dryden Wind Turbulence Model (Discrete (+q -r))1 : aerolibwind2/Dryden Wind Turbulence Model  (Continuous (+q -r))  units=Metric (MKS)  spec=MIL-F-8785C  model=Discrete Dryden (+q -r)  W20=10  Wdeg=0  TurbProb=10^-2 - Light  L_high=533.4  Wingspan=b_w*ft2m  ts=0.005  Seed=[23341 23342 23343 23344]  T_on=on
      settings: LibrarySourceBlock=|
      | aerolibwind2/Dryden Wind Turbulence Model
      | (Discrete (+q -r))
  Gain : Gain  Gain=-1
      settings: AttributesFormatString=Z to Alt
  Gain1 : Gain  Gain=ft2m
  Gain2 : Gain  Gain=m2ft
  Gain3 : Gain  Gain=-1
  Get Z : Selector  InputPortWidth=3  IndexOptions=Index vector (dialog)  Indices=[3]  OutputSizes=[(-2)]
  Product : Product  Multiplication=Matrix(*)
  Reduce Z Wind1 : Gain  Gain=[1 1 0.1]
      settings: AttributesFormatString=%<Gain>
  Rotation Angles to Direction Cosine Matrix : sharedtransform/Rotation Angles to Direction Cosine Matrix  rotationOrder=ZYX  aMode=aMode
  Selector : Selector  InputPortWidth=3  IndexOptions=Index vector (dialog)  Indices=[3 2 1]  OutputSizes=1
  Sqrt : Sqrt
  Terminator1 : Terminator
  Transfer Fcn : TransferFcn  Denominator=[0.02 1]
  Transfer Fcn1 : TransferFcn  Denominator=[0.02 1]
  Transpose : Math  Operator=transpose
  wind_b : Scope  NumInputPorts=3
  wind_e : Scope  NumInputPorts=3
  vb_wind : Outport  Unit=m/s  VectorParamsAs1DForOutWhenUnconnected=off
  wires:
  Euler/1 -> Selector/1
  Get Z/1 -> Transfer Fcn1/1
  Pe/1 -> Get Z/1
  Rotation Angles to Direction Cosine Matrix/1 -> Transpose/1, Dryden Wind Turbulence Model (Discrete (+q -r))1/3  "RECEF2B"
  Transfer Fcn1/1 -> Gain/1
  Transfer Fcn/1 -> Gain1/1
  Selector/1 -> Rotation Angles to Direction Cosine Matrix/1
  Reduce Z Wind1/1 -> Product/2, Gain2/1
  Dryden Wind Turbulence Model (Discrete (+q -r))1/1 -> Reduce Z Wind1/1
  Dryden Wind Turbulence Model (Discrete (+q -r))1/2 -> Terminator1/1
  Dot Product/1 -> Sqrt/1
  Sqrt/1 -> Transfer Fcn/1
  vb/1 -> Add/1, Dot Product/1, Dot Product/2
  Demux13/3 -> wind_b/3
  Demux13/2 -> wind_b/2
  Demux13/1 -> wind_b/1
  Gain/1 -> Dryden Wind Turbulence Model (Discrete (+q -r))1/1
  Add/1 -> vb_wind/1
  Gain1/1 -> Dryden Wind Turbulence Model (Discrete (+q -r))1/2
  Gain2/1 -> Demux13/1, Add/2
  Transpose/1 -> Product/1  "R_be"
  Product/1 -> Demux1/1
  Demux1/1 -> wind_e/1  "windex"
  Demux1/2 -> wind_e/2  "windey"
  Gain3/1 -> wind_e/3  "windez"
  Demux1/3 -> Gain3/1

== system TRUAV_Dynamics_from_GTRS_trim/Force and Moments/Gravity ==
  R_be : Inport
  Constant : Constant  Value=[0 0 32.2]'
  Demux : Demux  Outputs=3
  Matrix Multiply : Product  Multiplication=Matrix(*)
  Product7 : Product  Inputs=/  Multiplication=Matrix(*)
  Scope : Scope  NumInputPorts=3
  lbs : Gain  Gain=mass
  F_g : Outport
  wires:
  Matrix Multiply/1 -> lbs/1
  Constant/1 -> Matrix Multiply/2
  R_be/1 -> Product7/1
  lbs/1 -> Demux/1, F_g/1
  Demux/1 -> Scope/1
  Demux/2 -> Scope/2
  Demux/3 -> Scope/3
  Product7/1 -> Matrix Multiply/1  "DCM_be"

== system TRUAV_Dynamics_from_GTRS_trim/Force and Moments/Inertia moment and CG ==
  tiltangle : Inport
  Bus Selector : BusSelector  OutputSignals=Tilt1
  Constant : Constant  Value=[Ixx;Iyy; Izz; Ixz]
  Constant1 : Constant  Value=[pos_x_CG;pos_y_CG;pos_z_CG; pos_x_Nac; pos_y_Nac; pos_z_Nac;pos_x_H;pos_y_H;pos_z_H;L_n]
  Gain1 : Gain  Gain=[-20.5 -11.24 9.26 -1.76]
  MATLAB Function : MATLAB Function  TreatAsAtomicUnit=on
  Scope : Scope
  Sum : Sum  Inputs=|++
  gain_k_slugft_kgm1 : Gain  Gain=slugft2kgm
  rad2deg : Gain  Gain=rad2deg
  inertia moment : Outport
  CG : Outport  Port=2
  wires:
  Sum/1 -> Scope/1, inertia moment/1
  tiltangle/1 -> Bus Selector/1
  Bus Selector/1 -> MATLAB Function/1(beta_m), rad2deg/1  "<Tilt1>"
  rad2deg/1 -> Gain1/1
  Gain1/1 -> Sum/1
  Constant/1 -> Sum/2
  MATLAB Function/1(CG) -> CG/1
  Constant1/1 -> MATLAB Function/2(Pos)

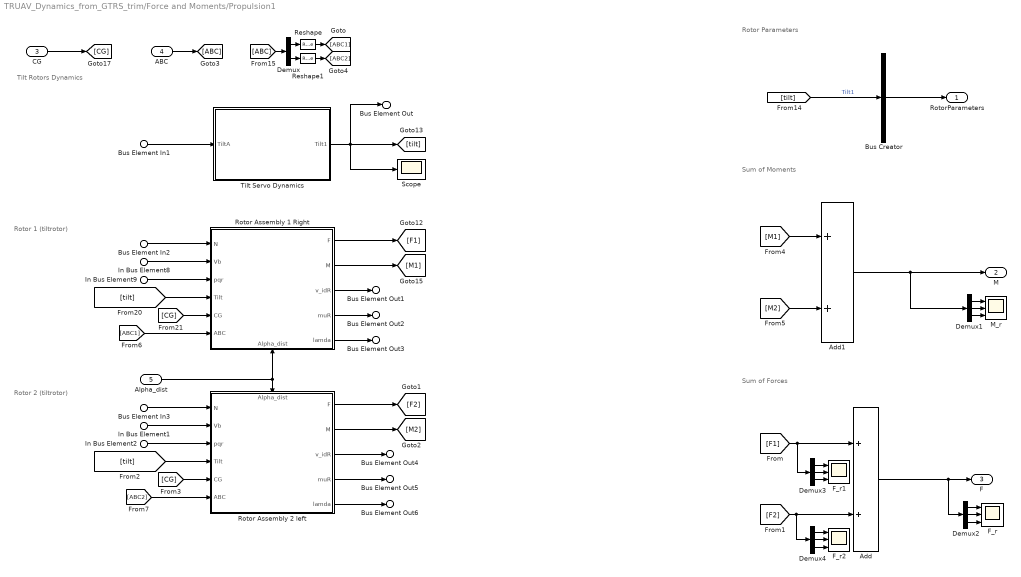
== system TRUAV_Dynamics_from_GTRS_trim/Force and Moments/Propulsion1 ==
  note: Rotor 2
      | (tiltrotor)
  note: Rotor 1
      | (tiltrotor)
  note: Rotor Parameters
  note: Sum of Forces
  note: Sum of Moments
  note: Tilt Rotors Dynamics
  Bus Element In2 : Inport  PortName=Actuator  Element=w1
  Bus Element In3 : Inport  PortName=Actuator  Element=w1
  Bus Element In1 : Inport  PortName=Actuator  Element=Tilt1
  In Bus Element8 : Inport  Port=2  PortName=States  Element=Vb
  In Bus Element1 : Inport  Port=2  PortName=States  Element=Vb
  In Bus Element9 : Inport  Port=2  PortName=States  Element=pqr
  In Bus Element2 : Inport  Port=2  PortName=States  Element=pqr
  CG : Inport  Port=3
  ABC : Inport  Port=4
  Alpha_dist : Inport  Port=5
  Add : Sum
  Add1 : Sum
  Bus Creator : BusCreator  Inputs=1
  Demux : Demux  Outputs=2
  Demux{1..4} (4 alike) : Demux  Outputs=3
  F_r : Scope  NumInputPorts=3
  F_r1 : Scope  NumInputPorts=3
  F_r2 : Scope  NumInputPorts=3
  M_r : Scope  NumInputPorts=3
  Reshape : Reshape  OutputDimensionality=Customize  OutputDimensions=[3,1]
  Reshape1 : Reshape  OutputDimensionality=Customize  OutputDimensions=[3,1]
  Rotor Assembly 1 Right : Subsystem
      settings: PortSchema="{\"entries\":[{\"content\":{\"sides\":[{\"content\":{\"connectorIds\":[\"In1\",\"In2\",\"In3\",\"In4\",\"In5\",\"In6\"]},\"type\":\"ConnectorPlacement.EquallySpacedRectSide\",\"uuid\":\"357592a5-cbc6-4fe3-abf9-44ec8c2897c1\"},{\"content\":{\"connectorIds\":[\"Out1\",\"Out2\",\"Out3\",\"Out4\",\"Out5\"],\"side\":\"RIGHT\"},\"type\":\"ConnectorPlacement.EquallySpacedRectSide\",\"uuid\":\"23cb046b-910e-4edf-a583-9c9760926d09\"},{\"content\":{\"connectorIds\":[],\"side\":\"TOP\"},\"type\":\"ConnectorPlacement.EquallySpacedRectSide\",\"uuid\":\"fa23253a-4b80-4716-8220-1eef7641310c\"},{\"content\":{\"connectorIds\":[\"In7\"],\"side\":\"BOTTOM\"},\"type\":\"ConnectorPlacement.EquallySpacedRectSide\",\"uuid\":\"706967b6-67f2-41ad-bbb6-e190ac646e87\"}]},\"type\":\"ConnectorPlacement.EquallySpacedConnector\",\"uuid\":\"4216a692-27ac-431a-a120-cbb862000bde\"}],\"packageUris\":[\"http://schema.mathworks.com/mf0/Connector/R2020b\"],\"version\":\"1.0\"}"
  Rotor Assembly 2 left : Subsystem
      settings: PortSchema="{\"entries\":[{\"content\":{\"sides\":[{\"content\":{\"connectorIds\":[\"In1\",\"In2\",\"In3\",\"In4\",\"In5\",\"In6\"]},\"type\":\"ConnectorPlacement.EquallySpacedRectSide\",\"uuid\":\"357592a5-cbc6-4fe3-abf9-44ec8c2897c1\"},{\"content\":{\"connectorIds\":[\"Out1\",\"Out2\",\"Out3\",\"Out4\",\"Out5\"],\"side\":\"RIGHT\"},\"type\":\"ConnectorPlacement.EquallySpacedRectSide\",\"uuid\":\"23cb046b-910e-4edf-a583-9c9760926d09\"},{\"content\":{\"connectorIds\":[\"In7\"],\"side\":\"TOP\"},\"type\":\"ConnectorPlacement.EquallySpacedRectSide\",\"uuid\":\"fa23253a-4b80-4716-8220-1eef7641310c\"}]},\"type\":\"ConnectorPlacement.EquallySpacedConnector\",\"uuid\":\"4216a692-27ac-431a-a120-cbb862000bde\"}],\"packageUris\":[\"http://schema.mathworks.com/mf0/Connector/R2020b\"],\"version\":\"1.0\"}"
  Scope : Scope
  Tilt Servo Dynamics : Subsystem
  RotorParameters : Outport
  M : Outport  Port=2
  F : Outport  Port=3
  Bus Element Out : Outport  Port=4  PortName=Rotor  Element=tilt
  Bus Element Out1 : Outport  Port=4  PortName=Rotor  Element=v_idR
  Bus Element Out2 : Outport  Port=4  PortName=Rotor  Element=muR
  Bus Element Out3 : Outport  Port=4  PortName=Rotor  Element=lamdaR
  Bus Element Out4 : Outport  Port=4  PortName=Rotor  Element=v_idL
  Bus Element Out5 : Outport  Port=4  PortName=Rotor  Element=muL
  Bus Element Out6 : Outport  Port=4  PortName=Rotor  Element=lamdaL
  wires:
  Rotor Assembly 2 left/4(muR) -> Bus Element Out5/1
  Rotor Assembly 2 left/3(v_idR) -> Bus Element Out4/1
  Tilt Servo Dynamics/1(Tilt1) -> Scope/1, [tilt], Bus Element Out/1
  Rotor Assembly 1 Right/5(lamda) -> Bus Element Out3/1
  Rotor Assembly 1 Right/4(muR) -> Bus Element Out2/1
  [ABC2] -> Rotor Assembly 2 left/6(ABC)
  [ABC1] -> Rotor Assembly 1 Right/6(ABC)
  Bus Element In3/1 -> Rotor Assembly 2 left/1(N)
  [tilt] -> Rotor Assembly 2 left/4(Tilt)
  In Bus Element2/1 -> Rotor Assembly 2 left/3(pqr)
  Rotor Assembly 2 left/2(M) -> [M2]
  Rotor Assembly 2 left/5(lamda) -> Bus Element Out6/1
  Rotor Assembly 2 left/1(F) -> [F2]
  In Bus Element1/1 -> Rotor Assembly 2 left/2(Vb)
  [CG] -> Rotor Assembly 2 left/5(CG)
  [CG] -> Rotor Assembly 1 Right/5(CG)
  CG/1 -> [CG]
  In Bus Element8/1 -> Rotor Assembly 1 Right/2(Vb)
  Rotor Assembly 1 Right/1(F) -> [F1]
  Rotor Assembly 1 Right/3(v_idR) -> Bus Element Out1/1
  Rotor Assembly 1 Right/2(M) -> [M1]
  In Bus Element9/1 -> Rotor Assembly 1 Right/3(pqr)
  [tilt] -> Rotor Assembly 1 Right/4(Tilt)
  Bus Element In2/1 -> Rotor Assembly 1 Right/1(N)
  Bus Element In1/1 -> Tilt Servo Dynamics/1(TiltA)
  [tilt] -> Bus Creator/1  "Tilt1"
  Bus Creator/1 -> RotorParameters/1
  [M1] -> Add1/1
  [M2] -> Add1/2
  [F1] -> Demux3/1, Add/1
  ABC/1 -> [ABC]
  [ABC] -> Demux/1
  Demux/1 -> Reshape/1
  Demux/2 -> Reshape1/1
  Reshape/1 -> [ABC1]
  Reshape1/1 -> [ABC2]
  Demux1/2 -> M_r/2
  Demux1/1 -> M_r/1
  Demux1/3 -> M_r/3
  Demux2/2 -> F_r/2
  Demux2/1 -> F_r/1
  Demux2/3 -> F_r/3
  Demux3/3 -> F_r1/3
  Demux3/1 -> F_r1/1
  Demux3/2 -> F_r1/2
  Demux4/3 -> F_r2/3
  Demux4/2 -> F_r2/2
  [F2] -> Demux4/1, Add/2
  Demux4/1 -> F_r2/1
  Add/1 -> Demux2/1, F/1
  Add1/1 -> Demux1/1, M/1
  Alpha_dist/1 -> Rotor Assembly 2 left/7(Alpha_dist), Rotor Assembly 1 Right/7(Alpha_dist)

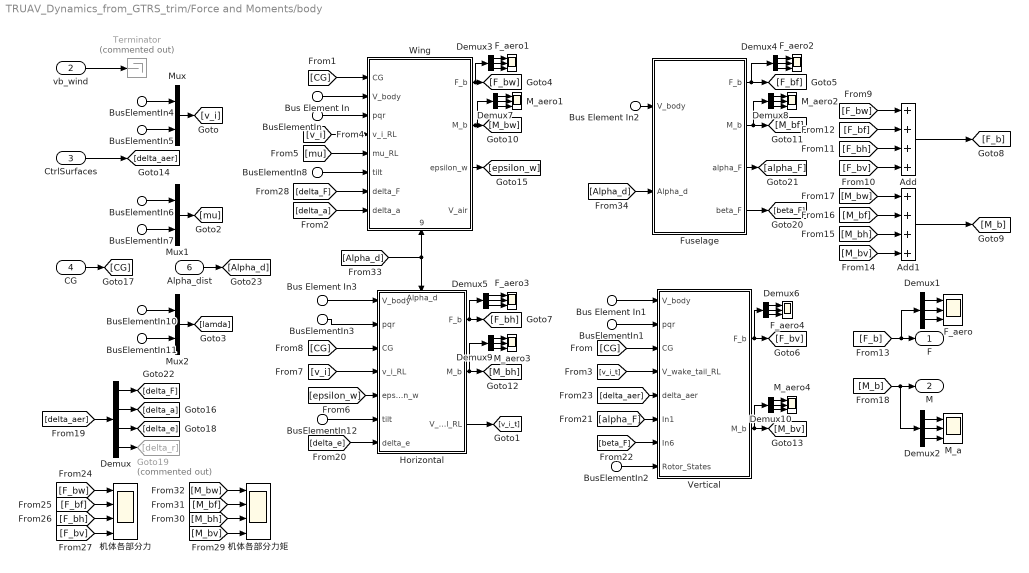
== system TRUAV_Dynamics_from_GTRS_trim/Force and Moments/body ==
  BusElementIn4 : Inport  PortName=Rotor_States  Element=v_idR
  BusElementIn6 : Inport  PortName=Rotor_States  Element=muR
  BusElementIn5 : Inport  PortName=Rotor_States  Element=v_idL
  BusElementIn7 : Inport  PortName=Rotor_States  Element=muL
  BusElementIn10 : Inport  PortName=Rotor_States  Element=lamdaR
  BusElementIn11 : Inport  PortName=Rotor_States  Element=lamdaL
  BusElementIn12 : Inport  PortName=Rotor_States  Element=tilt
  BusElementIn8 : Inport  PortName=Rotor_States  Element=tilt
  BusElementIn2 : Inport  PortName=Rotor_States  Element=tilt
  vb_wind : Inport  Port=2
  CtrlSurfaces : Inport  Port=3
  CG : Inport  Port=4
  Bus Element In{,1..3} (4 alike) : Inport  Port=5  PortName=States  Element=Vb
  BusElementIn : Inport  Port=5  PortName=States  Element=pqr
  BusElementIn1 : Inport  Port=5  PortName=States  Element=pqr
  BusElementIn3 : Inport  Port=5  PortName=States  Element=pqr
  Alpha_dist : Inport  Port=6
  Add : Sum  Inputs=++++
  Add1 : Sum  Inputs=++++
  Demux : Demux
  Demux{1..10} (10 alike) : Demux  Outputs=3
  F_aero{,1..4} (5 alike) : Scope  NumInputPorts=3
  Fuselage : Subsystem
  Goto19 : Goto  Commented=on  GotoTag=delta_r
  Horizontal : Subsystem
      settings: PortSchema="{\"entries\":[{\"content\":{\"sides\":[{\"content\":{\"connectorIds\":[\"In1\",\"In2\",\"In3\",\"In4\",\"In5\",\"In6\",\"In7\"]},\"type\":\"ConnectorPlacement.EquallySpacedRectSide\",\"uuid\":\"b1db04a2-6377-482b-ac13-d941978d34e1\"},{\"content\":{\"connectorIds\":[\"Out1\",\"Out2\",\"Out3\"],\"side\":\"RIGHT\"},\"type\":\"ConnectorPlacement.EquallySpacedRectSide\",\"uuid\":\"fb83f42f-2c69-4293-8d7c-1cbeac1f75cd\"},{\"content\":{\"connectorIds\":[\"In8\"],\"side\":\"TOP\"},\"type\":\"ConnectorPlacement.EquallySpacedRectSide\",\"uuid\":\"3d83034f-0725-4ce6-bb12-f11331056179\"}]},\"type\":\"ConnectorPlacement.EquallySpacedConnector\",\"uuid\":\"c5d4a0d2-fb15-4e1d-bef3-4dccd3d60521\"}],\"packageUris\":[\"http://schema.mathworks.com/mf0/Connector/R2020b\"],\"version\":\"1.0\"}"
  M_a : Scope  NumInputPorts=3
  M_aero{1..4} (4 alike) : Scope  NumInputPorts=3
  Mux : Mux  Inputs=2
  Mux1 : Mux  Inputs=2
  Mux2 : Mux  Inputs=2
  Terminator : Terminator  Commented=on
  Vertical : Subsystem
  Wing : Subsystem
      settings: PortSchema="{\"entries\":[{\"content\":{\"sides\":[{\"content\":{\"connectorIds\":[\"In1\",\"In2\",\"In3\",\"In4\",\"In5\",\"In6\",\"In7\",\"In8\"]},\"type\":\"ConnectorPlacement.EquallySpacedRectSide\",\"uuid\":\"91cdc459-7c0d-42af-9479-e6ce059298d3\"},{\"content\":{\"connectorIds\":[\"Out1\",\"Out2\",\"Out3\",\"Out4\"],\"side\":\"RIGHT\"},\"type\":\"ConnectorPlacement.EquallySpacedRectSide\",\"uuid\":\"d49a5f92-9f4b-4e2c-9533-fa0a930209c3\"},{\"content\":{\"connectorIds\":[],\"side\":\"TOP\"},\"type\":\"ConnectorPlacement.EquallySpacedRectSide\",\"uuid\":\"0d24c7fe-be7d-48e1-8ed4-a96e9f79a1d9\"},{\"content\":{\"connectorIds\":[\"In9\"],\"side\":\"BOTTOM\"},\"type\":\"ConnectorPlacement.EquallySpacedRectSide\",\"uuid\":\"3ca5ac7a-bb43-4b57-8132-e57a51e0e0f8\"}]},\"type\":\"ConnectorPlacement.EquallySpacedConnector\",\"uuid\":\"12283967-64d1-433d-87b9-06736187a2a5\"}],\"packageUris\":[\"http://schema.mathworks.com/mf0/Connector/R2020b\"],\"version\":\"1.0\"}"
  机体各部分力 : Scope  NumInputPorts=4
  机体各部分力矩 : Scope  NumInputPorts=4
  F : Outport
  M : Outport  Port=2
  wires:
  [M_bw] -> Add1/1
  [M_bf] -> Add1/2
  [M_bh] -> Add1/3
  [M_bv] -> Add1/4
  [F_b] -> Demux1/1, F/1
  [F_bv] -> Add/4
  [F_bh] -> Add/3
  [F_bf] -> Add/2
  [F_bw] -> Add/1
  Mux2/1 -> [lamda]
  BusElementIn11/1 -> Mux2/2
  BusElementIn10/1 -> Mux2/1
  BusElementIn6/1 -> Mux1/1
  BusElementIn7/1 -> Mux1/2
  Mux1/1 -> [mu]
  Mux/1 -> [v_i]
  BusElementIn5/1 -> Mux/2
  BusElementIn4/1 -> Mux/1
  CG/1 -> [CG]
  Bus Element In2/1 -> Fuselage/1(V_body)
  [CG] -> Wing/1(CG)
  Bus Element In/1 -> Wing/2(V_body)
  BusElementIn/1 -> Wing/3(pqr)
  [v_i] -> Wing/4(v_i_RL)
  [mu] -> Wing/5(mu_RL)
  BusElementIn8/1 -> Wing/6(tilt)
  Bus Element In3/1 -> Horizontal/1(V_body)
  BusElementIn3/1 -> Horizontal/2(pqr)
  [CG] -> Horizontal/3(CG)
  [v_i] -> Horizontal/4(v_i_RL)
  BusElementIn12/1 -> Horizontal/6(tilt)
  Horizontal/3(V_wake_tail_RL) -> [v_i_t]
  CtrlSurfaces/1 -> [delta_aer]
  [delta_a] -> Wing/8(delta_a)
  Wing/3(epsilon_w) -> [epsilon_w]
  [epsilon_w] -> Horizontal/5(epsilon_w)
  [delta_aer] -> Demux/1
  Demux/2 -> [delta_a]
  Demux/3 -> [delta_e]
  Demux/4 -> Goto19/1
  [delta_e] -> Horizontal/7(delta_e)
  Bus Element In1/1 -> Vertical/1(V_body)
  BusElementIn1/1 -> Vertical/2(pqr)
  [CG] -> Vertical/3(CG)
  [v_i_t] -> Vertical/4(V_wake_tail_RL)
  Vertical/1(F_b) -> Demux6/1, [F_bv]
  Vertical/2(M_b) -> Demux10/1, [M_bv]
  [delta_aer] -> Vertical/5(delta_aer)
  Fuselage/4(beta_F) -> [beta_F]
  [beta_F] -> Vertical/7(In6)
  BusElementIn2/1 -> Vertical/8(Rotor_States)
  Fuselage/3(alpha_F) -> [alpha_F]
  [alpha_F] -> Vertical/6(In1)
  [F_bw] -> 机体各部分力/1
  [F_bf] -> 机体各部分力/2
  [F_bh] -> 机体各部分力/3
  [F_bv] -> 机体各部分力/4
  Demux/1 -> [delta_F]
  [delta_F] -> Wing/7(delta_F)
  Add/1 -> [F_b]
  Add1/1 -> [M_b]
  Demux1/2 -> F_aero/2
  Demux1/1 -> F_aero/1
  Demux1/3 -> F_aero/3
  Demux2/1 -> M_a/1
  Demux2/2 -> M_a/2
  [M_b] -> Demux2/1, M/1
  Demux2/3 -> M_a/3
  [M_bw] -> 机体各部分力矩/1
  [M_bf] -> 机体各部分力矩/2
  [M_bh] -> 机体各部分力矩/3
  [M_bv] -> 机体各部分力矩/4
  Demux3/3 -> F_aero1/3
  Demux3/1 -> F_aero1/1
  Demux3/2 -> F_aero1/2
  Wing/1(F_b) -> [F_bw], Demux3/1
  Fuselage/1(F_b) -> Demux4/1, [F_bf]
  Demux4/2 -> F_aero2/2
  Demux4/1 -> F_aero2/1
  Demux4/3 -> F_aero2/3
  Demux5/1 -> F_aero3/1
  Demux5/2 -> F_aero3/2
  Horizontal/1(F_b) -> Demux5/1, [F_bh]
  Demux5/3 -> F_aero3/3
  Demux6/2 -> F_aero4/2
  Demux6/1 -> F_aero4/1
  Demux6/3 -> F_aero4/3
  [Alpha_d] -> Horizontal/8(Alpha_d), Wing/9(" ")
  Alpha_dist/1 -> [Alpha_d]
  [Alpha_d] -> Fuselage/2(Alpha_d)
  Wing/2(M_b) -> [M_bw], Demux7/1
  Demux7/2 -> M_aero1/2
  Demux7/1 -> M_aero1/1
  Demux7/3 -> M_aero1/3
  Demux8/3 -> M_aero2/3
  Demux8/1 -> M_aero2/1
  Demux8/2 -> M_aero2/2
  Fuselage/2(M_b) -> Demux8/1, [M_bf]
  Horizontal/2(M_b) -> Demux9/1, [M_bh]
  Demux9/2 -> M_aero3/2
  Demux9/1 -> M_aero3/1
  Demux9/3 -> M_aero3/3
  Demux10/3 -> M_aero4/3
  Demux10/1 -> M_aero4/1
  Demux10/2 -> M_aero4/2
  vb_wind/1 -> Terminator/1

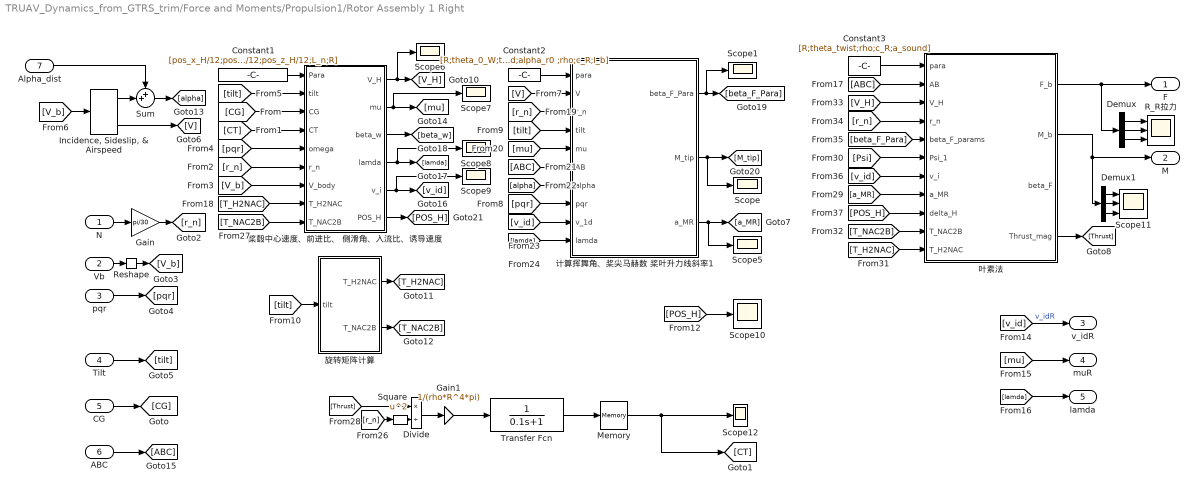
== system TRUAV_Dynamics_from_GTRS_trim/Force and Moments/Propulsion1/Rotor Assembly 1 Right ==
  N : Inport
  Vb : Inport  Port=2
  pqr : Inport  Port=3
  Tilt : Inport  Port=4
  CG : Inport  Port=5
  ABC : Inport  Port=6
  Alpha_dist : Inport  Port=7
  Constant1 : Constant  Value=[pos_x_H/12;pos_y_H/12;pos_z_H/12;L_n;R]
  Constant2 : Constant  Value=[R;theta_0_W;theta_0_R;theta_twist;a_sound;alpha_r0 ;rho;c_R;I_b]
  Constant3 : Constant  Value=[R;theta_twist;rho;c_R;a_sound]
  Demux : Demux  Outputs=3
  Demux1 : Demux  Outputs=3
  Divide : Product  Inputs=*/
  Gain : Gain  Gain=pi/30
  Gain1 : Gain  Gain=1/(rho*R^4*pi)
  "Incidence, Sideslip, & Airspeed" : aerolibasang/Incidence, Sideslip, & Airspeed
  Memory : Memory  InitialCondition=0.01
  R_R拉力 : Scope  NumInputPorts=3
  Reshape : Reshape  OutputDimensionality=Column vector (2-D)
  Scope{,1,5..10,12} (9 alike) : Scope
  Scope11 : Scope  NumInputPorts=3
  Square : Math  Operator=square
  Sum : Sum  Inputs=++|
  Transfer Fcn : TransferFcn  Denominator=[0.1 1]
  叶素法 : MATLAB Function  TreatAsAtomicUnit=on
  旋转矩阵计算 : MATLAB Function  TreatAsAtomicUnit=on
  桨毂中心速度、前进比、 侧滑角、入流比、诱导速度 : MATLAB Function  TreatAsAtomicUnit=on
  计算挥舞角、桨尖马赫数 桨叶升力线斜率1 : MATLAB Function  TreatAsAtomicUnit=on
  F : Outport
  M : Outport  Port=2
  v_idR : Outport  Port=3
  muR : Outport  Port=4
  lamda : Outport  Port=5
  wires:
  [ABC] -> 叶素法/2(AB)
  [mu] -> muR/1
  [lamda] -> lamda/1
  [v_id] -> v_idR/1  "v_idR"
  叶素法/1(F_b) -> F/1, Demux/1
  叶素法/2(M_b) -> Demux1/1, M/1
  [T_H2NAC] -> 叶素法/11(T_H2NAC)
  [T_NAC2B] -> 叶素法/10(T_NAC2B)
  [a_MR] -> 叶素法/8(a_MR)
  Constant3/1 -> 叶素法/1(para)
  [V_H] -> 叶素法/3(V_H)
  [r_n] -> 叶素法/4(r_n)
  [beta_F_Para] -> 叶素法/5(beta_F_params)
  [v_id] -> 叶素法/7(v_i)
  [POS_H] -> 叶素法/9(delta_H)
  ABC/1 -> [ABC]
  桨毂中心速度、前进比、 侧滑角、入流比、诱导速度/6(POS_H) -> [POS_H]
  计算挥舞角、桨尖马赫数 桨叶升力线斜率1/2(M_tip) -> Scope/1, [M_tip]
  计算挥舞角、桨尖马赫数 桨叶升力线斜率1/1(beta_F_Para) -> Scope1/1, [beta_F_Para]
  [lamda] -> 计算挥舞角、桨尖马赫数 桨叶升力线斜率1/10(lamda)
  桨毂中心速度、前进比、 侧滑角、入流比、诱导速度/4(lamda) -> Scope8/1, [lamda]
  [v_id] -> 计算挥舞角、桨尖马赫数 桨叶升力线斜率1/9(v_1d)
  桨毂中心速度、前进比、 侧滑角、入流比、诱导速度/5(v_i) -> Scope9/1, [v_id]
  [alpha] -> 计算挥舞角、桨尖马赫数 桨叶升力线斜率1/7(alpha)
  [ABC] -> 计算挥舞角、桨尖马赫数 桨叶升力线斜率1/6(AB)
  [mu] -> 计算挥舞角、桨尖马赫数 桨叶升力线斜率1/5(mu)
  [r_n] -> 计算挥舞角、桨尖马赫数 桨叶升力线斜率1/3(r_n)
  桨毂中心速度、前进比、 侧滑角、入流比、诱导速度/2(mu) -> Scope7/1, [mu]
  [T_H2NAC] -> 桨毂中心速度、前进比、 侧滑角、入流比、诱导速度/8(T_H2NAC)
  "Incidence, Sideslip, & Airspeed"/1 -> Sum/2
  旋转矩阵计算/2(T_NAC2B) -> [T_NAC2B]
  旋转矩阵计算/1(T_H2NAC) -> [T_H2NAC]
  [tilt] -> 旋转矩阵计算/1(tilt)
  桨毂中心速度、前进比、 侧滑角、入流比、诱导速度/1(V_H) -> Scope6/1, [V_H]
  [pqr] -> 计算挥舞角、桨尖马赫数 桨叶升力线斜率1/8(pqr)
  计算挥舞角、桨尖马赫数 桨叶升力线斜率1/3(a_MR) -> Scope5/1, [a_MR]
  Constant2/1 -> 计算挥舞角、桨尖马赫数 桨叶升力线斜率1/1(para)
  [tilt] -> 计算挥舞角、桨尖马赫数 桨叶升力线斜率1/4(tilt)
  [V] -> 计算挥舞角、桨尖马赫数 桨叶升力线斜率1/2(V)
  "Incidence, Sideslip, & Airspeed"/3 -> [V]
  [V_b] -> "Incidence, Sideslip, & Airspeed"/1
  [tilt] -> 桨毂中心速度、前进比、 侧滑角、入流比、诱导速度/2(tilt)
  Tilt/1 -> [tilt]
  [pqr] -> 桨毂中心速度、前进比、 侧滑角、入流比、诱导速度/5(omega)
  [V_b] -> 桨毂中心速度、前进比、 侧滑角、入流比、诱导速度/7(V_body)
  Vb/1 -> Reshape/1
  [r_n] -> 桨毂中心速度、前进比、 侧滑角、入流比、诱导速度/6(r_n)
  [CT] -> 桨毂中心速度、前进比、 侧滑角、入流比、诱导速度/4(CT)
  [CG] -> 桨毂中心速度、前进比、 侧滑角、入流比、诱导速度/3(CG)
  CG/1 -> [CG]
  Constant1/1 -> 桨毂中心速度、前进比、 侧滑角、入流比、诱导速度/1(Para)
  N/1 -> Gain/1
  pqr/1 -> [pqr]
  Gain/1 -> [r_n]
  [T_NAC2B] -> 桨毂中心速度、前进比、 侧滑角、入流比、诱导速度/9(T_NAC2B)
  [POS_H] -> Scope10/1
  Reshape/1 -> [V_b]
  桨毂中心速度、前进比、 侧滑角、入流比、诱导速度/3(beta_w) -> [beta_w]
  Memory/1 -> [CT], Scope12/1
  [Psi] -> 叶素法/6(Psi_1)
  Demux/1 -> R_R拉力/1
  Demux/2 -> R_R拉力/2
  Demux/3 -> R_R拉力/3
  Demux1/1 -> Scope11/1
  Demux1/2 -> Scope11/2
  Demux1/3 -> Scope11/3
  叶素法/4(Thrust_mag) -> [Thrust]
  [r_n] -> Square/1
  Transfer Fcn/1 -> Memory/1
  [Thrust] -> Divide/1
  Divide/1 -> Gain1/1
  Square/1 -> Divide/2
  Gain1/1 -> Transfer Fcn/1
  Sum/1 -> [alpha]
  Alpha_dist/1 -> Sum/1
